simulink model "RL_sus_quarter_sim"  (R2025a)
settings: Solver=FixedStepAuto  StartTime=0.0  StopTime=20  FixedStep=0.001  RelTol=1e-3
model workspace (MAT data in the model file):
  G0 : Simulink.Parameter (value not decoded)
  Q_F : Simulink.Parameter (value not decoded)
  Q_dot_s : Simulink.Parameter (value not decoded)
  Q_dot_s_h : Simulink.Parameter (value not decoded)
  Q_dot_u : Simulink.Parameter (value not decoded)
  Q_flec : Simulink.Parameter (value not decoded)
  Q_flec_t : Simulink.Parameter (value not decoded)
  b_deflec : Simulink.Parameter (value not decoded)
  bump_height : Simulink.Parameter (value not decoded)
  bump_lenth : Simulink.Parameter (value not decoded)
  bump_start : Simulink.Parameter (value not decoded)
  f0 : Simulink.Parameter (value not decoded)
  kt : Simulink.Parameter (value not decoded)
  ms : Simulink.Parameter (value not decoded)
  n0 : Simulink.Parameter (value not decoded)
  n1 : Simulink.Parameter (value not decoded)
  omega_1 : Simulink.Parameter (value not decoded)
  omega_2 : Simulink.Parameter (value not decoded)
  omega_3 : Simulink.Parameter (value not decoded)
  omega_4 : Simulink.Parameter (value not decoded)
  ramp_height : Simulink.Parameter (value not decoded)
  ramp_lenth : Simulink.Parameter (value not decoded)
  ramp_start : Simulink.Parameter (value not decoded)
  sine_amp : Simulink.Parameter (value not decoded)
  sine_freq : Simulink.Parameter (value not decoded)
  u : Simulink.Parameter (value not decoded)
symbols that are objects in the model workspace (value not decoded): b_deflec, bump_height, bump_lenth, bump_start, f0, G0, kt, ms, n0, n1, omega_1, omega_2, omega_3, omega_4, Q_dot_s, Q_dot_s_h, Q_F, Q_flec, Q_flec_t, ramp_height, ramp_lenth, ramp_start, sine_amp, sine_freq
undefined symbols (not defined in the file): Ground, Hook, SH_ADD_new_as_as_xdef
libraries: fl_lib x250, nesl_utility x48, sharedTrackingLibrary x34, dspstat3 x18, simulink x3, deeplib x2, slpidlib x1
(part 12 of 12)

== system RL_sus_quarter_sim/Quarter_sys/Control/Y_1/IFEKF freq c/Subsystem/MATLAB Function2/IFEKF simple ==
  y : Inport
  Constant : Constant  Value=diag([0,0,0,0,1])
  Constant7 : Constant  Value=10  SampleTime=0.001
  Extended Kalman Filter1 : sharedTrackingLibrary/Extended Kalman Filter  StateTransitionFcn=IFEKF_tfcn_simp  HasStateTransitionJacobianFcn=on  StateTransitionJacobianFcn=IFEKF_jcob_fcn_simp  HasAdditiveProcessNoise=Additive  ProcessNoise=[0,0,1e-7,1e-10,0]  HasTimeVaryingProcessNoise=on  HasStateTransitionFcnExtraArgument=0  InitialState=[0;-1;0;-1;0.1*pi;]  InitialStateCovariance=[1e-1,1e-1,1e-1,1e-1,1e-5]  MeasurementFcn1=IFEKF_measure_fcn_simp  HasMeasurementJacobianFcn1=on  MeasurementJacobianFcn1=IFEKF_mea_jcob_fcn_simp  HasMeasurementEnablePort1=off  HasAdditiveMeasurementNoise1=Additive  MeasurementNoise1=0.0001  HasTimeVaryingMeasurementNoise1=on  HasMeasurementFcnExtraArgument1=0  HasMeasurementWrapping1=off  MeasurementFcn2=myMeasurementFcn  HasMeasurementJacobianFcn2=off  HasMeasurementEnablePort2=off  HasAdditiveMeasurementNoise2=Additive  MeasurementNoise2=1  HasTimeVaryingMeasurementNoise2=off  HasMeasurementFcnExtraArgument2=0  HasMeasurementWrapping2=off  MeasurementFcn3=myMeasurementFcn  HasMeasurementJacobianFcn3=off  HasMeasurementEnablePort3=off  HasAdditiveMeasurementNoise3=Additive  MeasurementNoise3=1  HasTimeVaryingMeasurementNoise3=off  HasMeasurementFcnExtraArgument3=0  HasMeasurementWrapping3=off  MeasurementFcn4=myMeasurementFcn  HasMeasurementJacobianFcn4=off  HasMeasurementEnablePort4=off  HasAdditiveMeasurementNoise4=Additive  MeasurementNoise4=1  HasTimeVaryingMeasurementNoise4=off  HasMeasurementFcnExtraArgument4=0  HasMeasurementWrapping4=off  MeasurementFcn5=myMeasurementFcn  HasMeasurementJacobianFcn5=off  HasMeasurementEnablePort5=off  HasAdditiveMeasurementNoise5=Additive  MeasurementNoise5=1  HasTimeVaryingMeasurementNoise5=off  HasMeasurementFcnExtraArgument5=0  HasMeasurementWrapping5=off  EnableMultirate=off  StateTransitionFcnSampleTime=1  MeasurementFcn1SampleTime=1  MeasurementFcn2SampleTime=1  MeasurementFcn3SampleTime=1  MeasurementFcn4SampleTime=1  MeasurementFcn5SampleTime=1  UseCurrentEstimator=off  OutputStateCovariance=on  DataType=double  SampleTime=0.001  NumberOfMeasurements=1
  Gain6 : Gain  Gain=1/2/pi
  Scope1 : Scope
      settings: ActiveDisplayYMinimum=-108223.31295  ActiveDisplayYMaximum=120159.3313  DataLoggingVariableName=ScopeData2
  Scope6 : Scope
      settings: ActiveDisplayYMinimum=-5.04517  ActiveDisplayYMaximum=3.95687  DataLoggingVariableName=ScopeData3
  Selector1 : Selector  InputPortWidth=5  IndexOptions=Index vector (dialog)  Indices=[1]  OutputSizes=1
  Selector8 : Selector  InputPortWidth=5  IndexOptions=Index vector (dialog)  Indices=[5]  OutputSizes=1
  x1hat : Outport
  P : Outport  Port=2
  debug : Outport  Port=3
  xhat_pred : Outport  Port=4
  y_residual : Outport  Port=5
  omega : Outport  Port=6
  wires:
  y/1 -> Extended Kalman Filter1/2
  Extended Kalman Filter1/2 -> P/1
  Constant7/1 -> Extended Kalman Filter1/3
  Constant/1 -> Extended Kalman Filter1/1
  Gain6/1 -> omega/1, Scope6/1
  Selector8/1 -> Gain6/1
  Selector1/1 -> x1hat/1
  Extended Kalman Filter1/1 -> Selector1/1, Selector8/1, Scope1/1

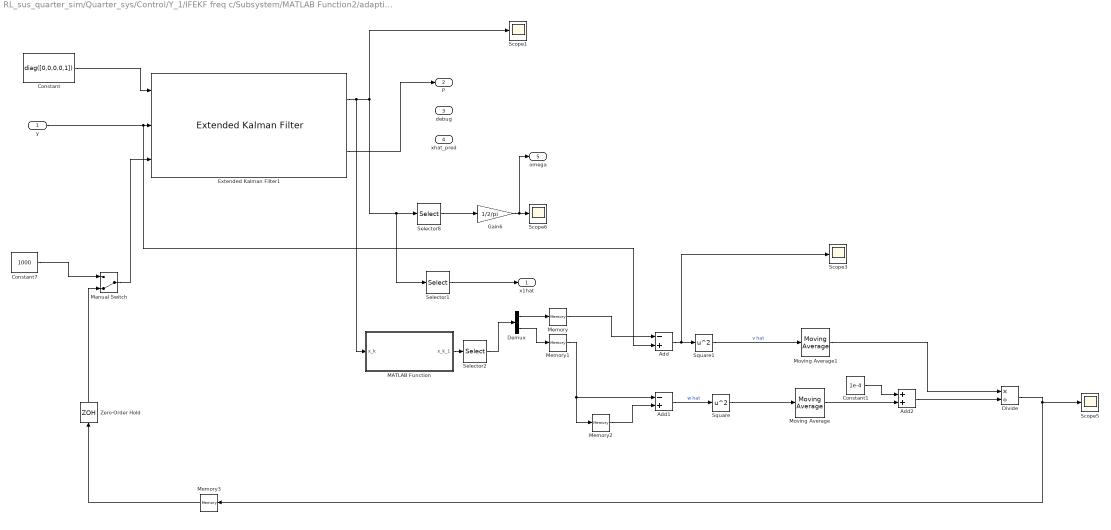
== system RL_sus_quarter_sim/Quarter_sys/Control/Y_1/IFEKF freq c/Subsystem/MATLAB Function2/adaptive IFEKF simple ==
  y : Inport
  Add : Sum  Inputs=-+
  Add1 : Sum  Inputs=-+
  Add2 : Sum
  Constant : Constant  Value=diag([0,0,0,0,1])
  Constant1 : Constant  Value=1e-4
  Constant7 : Constant  Value=1000  SampleTime=0.001
  Demux : Demux  Outputs=2
  Divide : Product  Inputs=*/
  Extended Kalman Filter1 : sharedTrackingLibrary/Extended Kalman Filter  StateTransitionFcn=IFEKF_tfcn_simp  HasStateTransitionJacobianFcn=on  StateTransitionJacobianFcn=IFEKF_jcob_fcn_simp  HasAdditiveProcessNoise=Additive  ProcessNoise=[0,0,1e-7,1e-10,0]  HasTimeVaryingProcessNoise=on  HasStateTransitionFcnExtraArgument=0  InitialState=[0;-1;0;-1;0.1*pi;]  InitialStateCovariance=[1e-1,1e-1,1e-1,1e-1,1e-5]  MeasurementFcn1=IFEKF_measure_fcn_simp  HasMeasurementJacobianFcn1=on  MeasurementJacobianFcn1=IFEKF_mea_jcob_fcn_simp  HasMeasurementEnablePort1=off  HasAdditiveMeasurementNoise1=Additive  MeasurementNoise1=0.0001  HasTimeVaryingMeasurementNoise1=on  HasMeasurementFcnExtraArgument1=0  HasMeasurementWrapping1=off  MeasurementFcn2=myMeasurementFcn  HasMeasurementJacobianFcn2=off  HasMeasurementEnablePort2=off  HasAdditiveMeasurementNoise2=Additive  MeasurementNoise2=1  HasTimeVaryingMeasurementNoise2=off  HasMeasurementFcnExtraArgument2=0  HasMeasurementWrapping2=off  MeasurementFcn3=myMeasurementFcn  HasMeasurementJacobianFcn3=off  HasMeasurementEnablePort3=off  HasAdditiveMeasurementNoise3=Additive  MeasurementNoise3=1  HasTimeVaryingMeasurementNoise3=off  HasMeasurementFcnExtraArgument3=0  HasMeasurementWrapping3=off  MeasurementFcn4=myMeasurementFcn  HasMeasurementJacobianFcn4=off  HasMeasurementEnablePort4=off  HasAdditiveMeasurementNoise4=Additive  MeasurementNoise4=1  HasTimeVaryingMeasurementNoise4=off  HasMeasurementFcnExtraArgument4=0  HasMeasurementWrapping4=off  MeasurementFcn5=myMeasurementFcn  HasMeasurementJacobianFcn5=off  HasMeasurementEnablePort5=off  HasAdditiveMeasurementNoise5=Additive  MeasurementNoise5=1  HasTimeVaryingMeasurementNoise5=off  HasMeasurementFcnExtraArgument5=0  HasMeasurementWrapping5=off  EnableMultirate=off  StateTransitionFcnSampleTime=1  MeasurementFcn1SampleTime=1  MeasurementFcn2SampleTime=1  MeasurementFcn3SampleTime=1  MeasurementFcn4SampleTime=1  MeasurementFcn5SampleTime=1  UseCurrentEstimator=off  OutputStateCovariance=on  DataType=double  SampleTime=0.001  NumberOfMeasurements=1
  Gain6 : Gain  Gain=1/2/pi
  MATLAB Function : MATLAB Function  TreatAsAtomicUnit=on
  Manual Switch : ManualSwitch  CurrentSetting=0
  Memory : Memory  InitialCondition=5
  Memory1 : Memory
  Memory2 : Memory  InitialCondition=1
  Memory3 : Memory  InitialCondition=10
  Moving Average : dspstat3/Moving Average  Method=Exponential weighting  ForgettingFactorPort=off  SpecifyWindowLength=off  WindowLength=100  OverlapLength=50  AllowArbitraryInputLength=on  ForgettingFactor=0.999  SimulateUsing=Interpreted execution
  Moving Average1 : dspstat3/Moving Average  Method=Exponential weighting  ForgettingFactorPort=off  SpecifyWindowLength=off  WindowLength=100  OverlapLength=50  AllowArbitraryInputLength=on  ForgettingFactor=0.999  SimulateUsing=Interpreted execution
  Scope{1,3,5..6} (4 alike) : Scope
      Scope1 settings: ActiveDisplayYMinimum=-108223.31295  ActiveDisplayYMaximum=120159.3313  DataLoggingVariableName=ScopeData3
      Scope3 settings: ActiveDisplayYMinimum=-5.93217  ActiveDisplayYMaximum=3.44712  DataLoggingVariableName=ScopeData4
      Scope5 settings: ActiveDisplayYMinimum=-180.87615  ActiveDisplayYMaximum=1627.8871  DataLoggingVariableName=ScopeData6
      Scope6 settings: ActiveDisplayYMinimum=-2.71822  ActiveDisplayYMaximum=5.24485  DataLoggingVariableName=ScopeData8
  Selector1 : Selector  InputPortWidth=5  IndexOptions=Index vector (dialog)  Indices=[1]  OutputSizes=1
  Selector2 : Selector  InputPortWidth=5  IndexOptions=Index vector (dialog)  Indices=[1 5]  OutputSizes=1
  Selector8 : Selector  InputPortWidth=5  IndexOptions=Index vector (dialog)  Indices=[5]  OutputSizes=1
  Square : Math  Operator=square
  Square1 : Math  Operator=square
  Zero-Order Hold : ZeroOrderHold  SampleTime=0.001
  x1hat : Outport
  P : Outport  Port=2
  debug : Outport  Port=3
  xhat_pred : Outport  Port=4
  omega : Outport  Port=5
  wires:
  Add1/1 -> Square/1  "w hat"
  Demux/2 -> Memory1/1
  Constant1/1 -> Add2/1
  Zero-Order Hold/1 -> Manual Switch/2
  Memory2/1 -> Add1/2
  Manual Switch/1 -> Extended Kalman Filter1/3
  MATLAB Function/1(x_k_1) -> Selector2/1
  Moving Average1/1 -> Divide/1
  Selector2/1 -> Demux/1
  Add2/1 -> Divide/2
  Constant/1 -> Extended Kalman Filter1/1
  Selector1/1 -> x1hat/1
  Moving Average/1 -> Add2/2
  Memory/1 -> Add/1
  Extended Kalman Filter1/1 -> MATLAB Function/1(x_k), Scope1/1, Selector8/1, Selector1/1
  y/1 -> Add/2, Extended Kalman Filter1/2
  Memory1/1 -> Add1/1, Memory2/1
  Square/1 -> Moving Average/1
  Square1/1 -> Moving Average1/1  "v hat"
  Extended Kalman Filter1/2 -> P/1
  Divide/1 -> Memory3/1, Scope5/1
  Selector8/1 -> Gain6/1
  Demux/1 -> Memory/1
  Add/1 -> Scope3/1, Square1/1
  Memory3/1 -> Zero-Order Hold/1
  Gain6/1 -> Scope6/1, omega/1
  Constant7/1 -> Manual Switch/1

== system RL_sus_quarter_sim/Quarter_sys/Control/Y_1/imp_force_RL_model/Subsystem/MATLAB Function2/EKF epsilon ==
  y : Inport
  epsilon : Inport  Port=2
  Constant : Constant  Value=diag([0,0,1,0])
  Constant7 : Constant  Value=500  SampleTime=0.001
  Extended Kalman Filter1 : sharedTrackingLibrary/Extended Kalman Filter  StateTransitionFcn=IFEKF_tfcn_ep  HasStateTransitionJacobianFcn=on  StateTransitionJacobianFcn=IFEKF_jcob_fcn_ep  HasAdditiveProcessNoise=Additive  ProcessNoise=[0,0,1e-7,1e-10]  HasTimeVaryingProcessNoise=on  HasStateTransitionFcnExtraArgument=1  InitialState=[0;-0.2;1*2*pi;0.2;]  InitialStateCovariance=[1e-1,1e-1,1e-1,1e-5]  MeasurementFcn1=IFEKF_measure_fcn_mod  HasMeasurementJacobianFcn1=on  MeasurementJacobianFcn1=IFEKF_mea_jcob_fcn_mod  HasMeasurementEnablePort1=off  HasAdditiveMeasurementNoise1=Additive  MeasurementNoise1=0.0001  HasTimeVaryingMeasurementNoise1=on  HasMeasurementFcnExtraArgument1=0  HasMeasurementWrapping1=off  MeasurementFcn2=myMeasurementFcn  HasMeasurementJacobianFcn2=off  HasMeasurementEnablePort2=off  HasAdditiveMeasurementNoise2=Additive  MeasurementNoise2=1  HasTimeVaryingMeasurementNoise2=off  HasMeasurementFcnExtraArgument2=0  HasMeasurementWrapping2=off  MeasurementFcn3=myMeasurementFcn  HasMeasurementJacobianFcn3=off  HasMeasurementEnablePort3=off  HasAdditiveMeasurementNoise3=Additive  MeasurementNoise3=1  HasTimeVaryingMeasurementNoise3=off  HasMeasurementFcnExtraArgument3=0  HasMeasurementWrapping3=off  MeasurementFcn4=myMeasurementFcn  HasMeasurementJacobianFcn4=off  HasMeasurementEnablePort4=off  HasAdditiveMeasurementNoise4=Additive  MeasurementNoise4=1  HasTimeVaryingMeasurementNoise4=off  HasMeasurementFcnExtraArgument4=0  HasMeasurementWrapping4=off  MeasurementFcn5=myMeasurementFcn  HasMeasurementJacobianFcn5=off  HasMeasurementEnablePort5=off  HasAdditiveMeasurementNoise5=Additive  MeasurementNoise5=1  HasTimeVaryingMeasurementNoise5=off  HasMeasurementFcnExtraArgument5=0  HasMeasurementWrapping5=off  EnableMultirate=off  StateTransitionFcnSampleTime=1  MeasurementFcn1SampleTime=1  MeasurementFcn2SampleTime=1  MeasurementFcn3SampleTime=1  MeasurementFcn4SampleTime=1  MeasurementFcn5SampleTime=1  UseCurrentEstimator=off  OutputStateCovariance=on  DataType=double  SampleTime=0.001  NumberOfMeasurements=1
  Gain6 : Gain  Gain=1/2/pi
  Scope6 : Scope
      settings: ActiveDisplayYMinimum=-0.3996  ActiveDisplayYMaximum=6.53697  DataLoggingVariableName=ScopeData2
  Selector1 : Selector  InputPortWidth=4  IndexOptions=Index vector (dialog)  Indices=[1]  OutputSizes=1
  Selector8 : Selector  InputPortWidth=4  IndexOptions=Index vector (dialog)  Indices=[3]  OutputSizes=1
  x1hat : Outport
  P : Outport  Port=2
  debug : Outport  Port=3
  xhat_pred : Outport  Port=4
  y_residual : Outport  Port=5
  omega : Outport  Port=6
  wires:
  y/1 -> Extended Kalman Filter1/3
  Extended Kalman Filter1/2 -> P/1
  Constant7/1 -> Extended Kalman Filter1/4
  epsilon/1 -> Extended Kalman Filter1/2
  Constant/1 -> Extended Kalman Filter1/1
  Gain6/1 -> omega/1, Scope6/1
  Selector8/1 -> Gain6/1
  Extended Kalman Filter1/1 -> Selector1/1, Selector8/1
  Selector1/1 -> x1hat/1

== system RL_sus_quarter_sim/Quarter_sys/Control/Y_1/imp_force_RL_model/Subsystem/MATLAB Function2/EKF simple Amp ==
  y : Inport
  epsilon : Inport  Port=2
  Constant5 : Constant  Value=0.1e-5
  Constant7 : Constant  Value=0.11  SampleTime=0.001
  Extended Kalman Filter1 : sharedTrackingLibrary/Extended Kalman Filter  StateTransitionFcn=IFEKF_tfcn_amp  HasStateTransitionJacobianFcn=on  StateTransitionJacobianFcn=IFEKF_jcob_fcn_amp  HasAdditiveProcessNoise=Additive  ProcessNoise=[0,0,1e-7,1e-10]  HasTimeVaryingProcessNoise=on  HasStateTransitionFcnExtraArgument=1  InitialState=[0;-0.5;2*pi;0.5;]  InitialStateCovariance=[1e-1,1e-1,1e-1,1e-5]  MeasurementFcn1=IFEKF_measure_fcn_amp  HasMeasurementJacobianFcn1=on  MeasurementJacobianFcn1=IFEKF_mea_jcob_fcn_amp  HasMeasurementEnablePort1=off  HasAdditiveMeasurementNoise1=Additive  MeasurementNoise1=0.0001  HasTimeVaryingMeasurementNoise1=on  HasMeasurementFcnExtraArgument1=0  HasMeasurementWrapping1=off  MeasurementFcn2=myMeasurementFcn  HasMeasurementJacobianFcn2=off  HasMeasurementEnablePort2=off  HasAdditiveMeasurementNoise2=Additive  MeasurementNoise2=1  HasTimeVaryingMeasurementNoise2=off  HasMeasurementFcnExtraArgument2=0  HasMeasurementWrapping2=off  MeasurementFcn3=myMeasurementFcn  HasMeasurementJacobianFcn3=off  HasMeasurementEnablePort3=off  HasAdditiveMeasurementNoise3=Additive  MeasurementNoise3=1  HasTimeVaryingMeasurementNoise3=off  HasMeasurementFcnExtraArgument3=0  HasMeasurementWrapping3=off  MeasurementFcn4=myMeasurementFcn  HasMeasurementJacobianFcn4=off  HasMeasurementEnablePort4=off  HasAdditiveMeasurementNoise4=Additive  MeasurementNoise4=1  HasTimeVaryingMeasurementNoise4=off  HasMeasurementFcnExtraArgument4=0  HasMeasurementWrapping4=off  MeasurementFcn5=myMeasurementFcn  HasMeasurementJacobianFcn5=off  HasMeasurementEnablePort5=off  HasAdditiveMeasurementNoise5=Additive  MeasurementNoise5=1  HasTimeVaryingMeasurementNoise5=off  HasMeasurementFcnExtraArgument5=0  HasMeasurementWrapping5=off  EnableMultirate=off  StateTransitionFcnSampleTime=1  MeasurementFcn1SampleTime=1  MeasurementFcn2SampleTime=1  MeasurementFcn3SampleTime=1  MeasurementFcn4SampleTime=1  MeasurementFcn5SampleTime=1  UseCurrentEstimator=off  OutputStateCovariance=on  DataType=double  SampleTime=0.001  NumberOfMeasurements=1
  Gain6 : Gain  Gain=1/2/pi
  MATLAB Function : MATLAB Function
  Scope1 : Scope
      settings: ActiveDisplayYMinimum=-1.3479  ActiveDisplayYMaximum=7.13108  DataLoggingVariableName=ScopeData7
  Scope6 : Scope
      settings: ActiveDisplayYMinimum=0.9999988  ActiveDisplayYMaximum=1.0000001
  Selector1 : Selector  InputPortWidth=4  IndexOptions=Index vector (dialog)  Indices=[1]  OutputSizes=1
  Selector8 : Selector  InputPortWidth=4  IndexOptions=Index vector (dialog)  Indices=[3]  OutputSizes=1
  x1hat : Outport
  P : Outport  Port=2
  debug : Outport  Port=3
  xhat_pred : Outport  Port=4
  y_residual : Outport  Port=5
  omega : Outport  Port=6
  wires:
  epsilon/1 -> Extended Kalman Filter1/2
  Constant7/1 -> Extended Kalman Filter1/4
  Constant5/1 -> MATLAB Function/1(gamma)
  Extended Kalman Filter1/2 -> P/1
  y/1 -> Extended Kalman Filter1/3
  MATLAB Function/1(y) -> Extended Kalman Filter1/1
  Extended Kalman Filter1/1 -> Selector1/1, Selector8/1, Scope1/1
  Selector8/1 -> Gain6/1
  Gain6/1 -> omega/1, Scope6/1
  Selector1/1 -> x1hat/1

== system RL_sus_quarter_sim/Quarter_sys/Control/Y_1/imp_force_RL_model/Subsystem/MATLAB Function2/IFEKF simple ==
  y : Inport
  Constant : Constant  Value=diag([0,0,0,0,1])
  Constant7 : Constant  Value=10  SampleTime=0.001
  Extended Kalman Filter1 : sharedTrackingLibrary/Extended Kalman Filter  StateTransitionFcn=IFEKF_tfcn_simp  HasStateTransitionJacobianFcn=on  StateTransitionJacobianFcn=IFEKF_jcob_fcn_simp  HasAdditiveProcessNoise=Additive  ProcessNoise=[0,0,1e-7,1e-10,0]  HasTimeVaryingProcessNoise=on  HasStateTransitionFcnExtraArgument=0  InitialState=[0;-1;0;-1;0.1*pi;]  InitialStateCovariance=[1e-1,1e-1,1e-1,1e-1,1e-5]  MeasurementFcn1=IFEKF_measure_fcn_simp  HasMeasurementJacobianFcn1=on  MeasurementJacobianFcn1=IFEKF_mea_jcob_fcn_simp  HasMeasurementEnablePort1=off  HasAdditiveMeasurementNoise1=Additive  MeasurementNoise1=0.0001  HasTimeVaryingMeasurementNoise1=on  HasMeasurementFcnExtraArgument1=0  HasMeasurementWrapping1=off  MeasurementFcn2=myMeasurementFcn  HasMeasurementJacobianFcn2=off  HasMeasurementEnablePort2=off  HasAdditiveMeasurementNoise2=Additive  MeasurementNoise2=1  HasTimeVaryingMeasurementNoise2=off  HasMeasurementFcnExtraArgument2=0  HasMeasurementWrapping2=off  MeasurementFcn3=myMeasurementFcn  HasMeasurementJacobianFcn3=off  HasMeasurementEnablePort3=off  HasAdditiveMeasurementNoise3=Additive  MeasurementNoise3=1  HasTimeVaryingMeasurementNoise3=off  HasMeasurementFcnExtraArgument3=0  HasMeasurementWrapping3=off  MeasurementFcn4=myMeasurementFcn  HasMeasurementJacobianFcn4=off  HasMeasurementEnablePort4=off  HasAdditiveMeasurementNoise4=Additive  MeasurementNoise4=1  HasTimeVaryingMeasurementNoise4=off  HasMeasurementFcnExtraArgument4=0  HasMeasurementWrapping4=off  MeasurementFcn5=myMeasurementFcn  HasMeasurementJacobianFcn5=off  HasMeasurementEnablePort5=off  HasAdditiveMeasurementNoise5=Additive  MeasurementNoise5=1  HasTimeVaryingMeasurementNoise5=off  HasMeasurementFcnExtraArgument5=0  HasMeasurementWrapping5=off  EnableMultirate=off  StateTransitionFcnSampleTime=1  MeasurementFcn1SampleTime=1  MeasurementFcn2SampleTime=1  MeasurementFcn3SampleTime=1  MeasurementFcn4SampleTime=1  MeasurementFcn5SampleTime=1  UseCurrentEstimator=off  OutputStateCovariance=on  DataType=double  SampleTime=0.001  NumberOfMeasurements=1
  Gain6 : Gain  Gain=1/2/pi
  Scope1 : Scope
      settings: ActiveDisplayYMinimum=-108223.31295  ActiveDisplayYMaximum=120159.3313  DataLoggingVariableName=ScopeData2
  Scope6 : Scope
      settings: ActiveDisplayYMinimum=-5.04517  ActiveDisplayYMaximum=3.95687  DataLoggingVariableName=ScopeData3
  Selector1 : Selector  InputPortWidth=5  IndexOptions=Index vector (dialog)  Indices=[1]  OutputSizes=1
  Selector8 : Selector  InputPortWidth=5  IndexOptions=Index vector (dialog)  Indices=[5]  OutputSizes=1
  x1hat : Outport
  P : Outport  Port=2
  debug : Outport  Port=3
  xhat_pred : Outport  Port=4
  y_residual : Outport  Port=5
  omega : Outport  Port=6
  wires:
  y/1 -> Extended Kalman Filter1/2
  Extended Kalman Filter1/2 -> P/1
  Constant7/1 -> Extended Kalman Filter1/3
  Constant/1 -> Extended Kalman Filter1/1
  Gain6/1 -> omega/1, Scope6/1
  Selector8/1 -> Gain6/1
  Selector1/1 -> x1hat/1
  Extended Kalman Filter1/1 -> Selector1/1, Selector8/1, Scope1/1

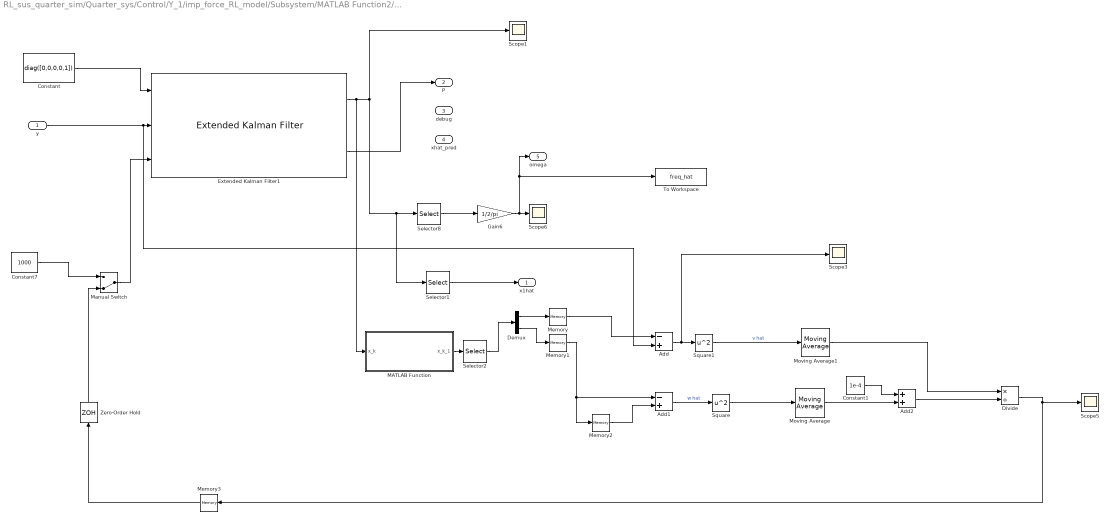
== system RL_sus_quarter_sim/Quarter_sys/Control/Y_1/imp_force_RL_model/Subsystem/MATLAB Function2/adaptive IFEKF simple ==
  y : Inport
  Add : Sum  Inputs=-+
  Add1 : Sum  Inputs=-+
  Add2 : Sum
  Constant : Constant  Value=diag([0,0,0,0,1])
  Constant1 : Constant  Value=1e-4
  Constant7 : Constant  Value=1000  SampleTime=0.001
  Demux : Demux  Outputs=2
  Divide : Product  Inputs=*/
  Extended Kalman Filter1 : sharedTrackingLibrary/Extended Kalman Filter  StateTransitionFcn=IFEKF_tfcn_simp  HasStateTransitionJacobianFcn=on  StateTransitionJacobianFcn=IFEKF_jcob_fcn_simp  HasAdditiveProcessNoise=Additive  ProcessNoise=[0,0,1e-7,1e-10,0]  HasTimeVaryingProcessNoise=on  HasStateTransitionFcnExtraArgument=0  InitialState=[0;-1;0;-1;0.1*pi;]  InitialStateCovariance=[1e-1,1e-1,1e-1,1e-1,1e-5]  MeasurementFcn1=IFEKF_measure_fcn_simp  HasMeasurementJacobianFcn1=on  MeasurementJacobianFcn1=IFEKF_mea_jcob_fcn_simp  HasMeasurementEnablePort1=off  HasAdditiveMeasurementNoise1=Additive  MeasurementNoise1=0.0001  HasTimeVaryingMeasurementNoise1=on  HasMeasurementFcnExtraArgument1=0  HasMeasurementWrapping1=off  MeasurementFcn2=myMeasurementFcn  HasMeasurementJacobianFcn2=off  HasMeasurementEnablePort2=off  HasAdditiveMeasurementNoise2=Additive  MeasurementNoise2=1  HasTimeVaryingMeasurementNoise2=off  HasMeasurementFcnExtraArgument2=0  HasMeasurementWrapping2=off  MeasurementFcn3=myMeasurementFcn  HasMeasurementJacobianFcn3=off  HasMeasurementEnablePort3=off  HasAdditiveMeasurementNoise3=Additive  MeasurementNoise3=1  HasTimeVaryingMeasurementNoise3=off  HasMeasurementFcnExtraArgument3=0  HasMeasurementWrapping3=off  MeasurementFcn4=myMeasurementFcn  HasMeasurementJacobianFcn4=off  HasMeasurementEnablePort4=off  HasAdditiveMeasurementNoise4=Additive  MeasurementNoise4=1  HasTimeVaryingMeasurementNoise4=off  HasMeasurementFcnExtraArgument4=0  HasMeasurementWrapping4=off  MeasurementFcn5=myMeasurementFcn  HasMeasurementJacobianFcn5=off  HasMeasurementEnablePort5=off  HasAdditiveMeasurementNoise5=Additive  MeasurementNoise5=1  HasTimeVaryingMeasurementNoise5=off  HasMeasurementFcnExtraArgument5=0  HasMeasurementWrapping5=off  EnableMultirate=off  StateTransitionFcnSampleTime=1  MeasurementFcn1SampleTime=1  MeasurementFcn2SampleTime=1  MeasurementFcn3SampleTime=1  MeasurementFcn4SampleTime=1  MeasurementFcn5SampleTime=1  UseCurrentEstimator=off  OutputStateCovariance=on  DataType=double  SampleTime=0.001  NumberOfMeasurements=1
  Gain6 : Gain  Gain=1/2/pi
  MATLAB Function : MATLAB Function  TreatAsAtomicUnit=on
  Manual Switch : ManualSwitch  CurrentSetting=0
  Memory : Memory  InitialCondition=5
  Memory1 : Memory
  Memory2 : Memory  InitialCondition=1
  Memory3 : Memory  InitialCondition=10
  Moving Average : dspstat3/Moving Average  Method=Exponential weighting  ForgettingFactorPort=off  SpecifyWindowLength=off  WindowLength=100  OverlapLength=50  AllowArbitraryInputLength=on  ForgettingFactor=0.999  SimulateUsing=Interpreted execution
  Moving Average1 : dspstat3/Moving Average  Method=Exponential weighting  ForgettingFactorPort=off  SpecifyWindowLength=off  WindowLength=100  OverlapLength=50  AllowArbitraryInputLength=on  ForgettingFactor=0.999  SimulateUsing=Interpreted execution
  Scope{1,3,5..6} (4 alike) : Scope
      Scope1 settings: ActiveDisplayYMinimum=-5.9836760801118811E+37  ActiveDisplayYMaximum=5.3206752918754988E+37  DataLoggingVariableName=ScopeData3
      Scope3 settings: ActiveDisplayYMinimum=-5.93217  ActiveDisplayYMaximum=3.44712  DataLoggingVariableName=ScopeData4
      Scope5 settings: ActiveDisplayYMinimum=-182.59879  ActiveDisplayYMaximum=1643.39044  DataLoggingVariableName=ScopeData6
      Scope6 settings: ActiveDisplayYMinimum=-3.1891  ActiveDisplayYMaximum=3.16461  DataLoggingVariableName=ScopeData8
  Selector1 : Selector  InputPortWidth=5  IndexOptions=Index vector (dialog)  Indices=[1]  OutputSizes=1
  Selector2 : Selector  InputPortWidth=5  IndexOptions=Index vector (dialog)  Indices=[1 5]  OutputSizes=1
  Selector8 : Selector  InputPortWidth=5  IndexOptions=Index vector (dialog)  Indices=[5]  OutputSizes=1
  Square : Math  Operator=square
  Square1 : Math  Operator=square
  To Workspace : ToWorkspace  VariableName=freq_hat  SampleTime=-1
  Zero-Order Hold : ZeroOrderHold  SampleTime=0.001
  x1hat : Outport
  P : Outport  Port=2
  debug : Outport  Port=3
  xhat_pred : Outport  Port=4
  omega : Outport  Port=5
  wires:
  Add1/1 -> Square/1  "w hat"
  Demux/2 -> Memory1/1
  Constant1/1 -> Add2/1
  Zero-Order Hold/1 -> Manual Switch/2
  Memory2/1 -> Add1/2
  Manual Switch/1 -> Extended Kalman Filter1/3
  MATLAB Function/1(x_k_1) -> Selector2/1
  Moving Average1/1 -> Divide/1
  Selector2/1 -> Demux/1
  Add2/1 -> Divide/2
  Constant/1 -> Extended Kalman Filter1/1
  Selector1/1 -> x1hat/1
  Moving Average/1 -> Add2/2
  Memory/1 -> Add/1
  Extended Kalman Filter1/1 -> MATLAB Function/1(x_k), Scope1/1, Selector8/1, Selector1/1
  y/1 -> Add/2, Extended Kalman Filter1/2
  Memory1/1 -> Add1/1, Memory2/1
  Square/1 -> Moving Average/1
  Square1/1 -> Moving Average1/1  "v hat"
  Extended Kalman Filter1/2 -> P/1
  Divide/1 -> Memory3/1, Scope5/1
  Selector8/1 -> Gain6/1
  Demux/1 -> Memory/1
  Add/1 -> Scope3/1, Square1/1
  Memory3/1 -> Zero-Order Hold/1
  Gain6/1 -> Scope6/1, To Workspace/1, omega/1
  Constant7/1 -> Manual Switch/1

== matlab function RL_sus_quarter_sim/road_profile/gp/MATLAB Function ==
  data: X input; u output; gp_sample input; x input
function u = u_fn(X, gp_sample, x)
    u = interp1(X, gp_sample, x, 'linear', 'extrap');
end

== matlab function RL_sus_quarter_sim/Quarter_sys/Control/Y_1/SH_ADD_new_as_as_xdef^2/2nd_FS_adef_vs/MATLAB Function1 ==
  data: as input; xdef input; y output; alpha input; ks input; ms input; cs input
function y = fcn(as,xdef,alpha,ks,ms,cs)

H2 = (cs^4*alpha^4 + (2*cs^2*ks^2)*alpha^2 + ks^4)/(ms^4*alpha^2);
y = xdef^4/as^2* alpha^2 * H2;

end

== matlab function RL_sus_quarter_sim/Quarter_sys/Control/Y_1/IFEKF freq bkkcc/Subsystem/MATLAB Function2/EKF simple Amp/MATLAB Function ==
  data: gamma input; y output size=[4,4]
function y = fcn(gamma)
% u = [0;0;gamma;1];
u = [0;0;1;gamma];
y = diag(u);
end

== matlab function RL_sus_quarter_sim/Quarter_sys/Control/Y_1/IFEKF freq bkkcc/Subsystem/MATLAB Function2/adaptive IFEKF simple/MATLAB Function ==
  data: x_k input; x_k_1 output
function x_k_1 = IFEKF_tfcn_simp(x_k)
x_k_1 = zeros(5,1);
dt = 0.001;
x_k_1(1) = 2*cos(x_k(5)*dt) * x_k(1) - x_k(2) ;
x_k_1(2) = x_k(1);
x_k_1(3) = 2*cos(x_k(5)*dt) * x_k(3) - x_k(4);
x_k_1(4) = x_k(3);
x_k_1(5) = x_k(5);
 
end

== stateflow chart RL_sus_quarter_sim/Quarter_sys/Control/Y_1/IFEKF freq bkkcc/Subsystem/Chart ==
  state L2
    entry:count = 0;
    level = 2;
    during:count = count+1;
    level = 2;
  state L1
    entry:count = 0;
    level = 1;
    during:count = count+1;
    level = 1;
  (default) -> L1
  L1 -> L2 : [freq > (FS1+0.1)&&freq<(FS2-0.1)&&count>=100]
  L2 -> L1 : [(freq<(FS1-0.1)&&count>=100)||(freq>(FS2+0.1)&&count>=100)]
  data: freq input; level output; FS1 input; FS2 input; data local; count local

== stateflow chart RL_sus_quarter_sim/Quarter_sys/Control/Y_1/imp_force_RL_model/Subsystem/Chart ==
  state L2
    entry:count = 0;
    level = 2;
    during:count = count+1;
    level = 2;
  state L1
    entry:count = 0;
    level = 1;
    during:count = count+1;
    level = 1;
  (default) -> L1
  L1 -> L2 : [freq > (FS1+0.1)&&freq<(FS2-0.1)&&count>=100]
  L2 -> L1 : [(freq<(FS1-0.1)&&count>=100)||(freq>(FS2+0.1)&&count>=100)]
  data: freq input; level output; FS1 input; FS2 input; data local; count local

== matlab function RL_sus_quarter_sim/Quarter_sys/Control/Y_1/IFEKF SHADD/Subsystem/MATLAB Function ==
  data: u input; FS_1 input; y output; FS_2 input; FS_3 input
function y = fcn(u,FS_1,FS_2,FS_3)

    % if u < FS_1
    %     y = 3;
    % elseif u >= FS_1 && u < FS_2
    %     y = 1;
    % elseif u >= FS_2 && u < FS_3
    %     y = 2;
    % else
    %     y = 1;
    % end


    if u < FS_1
        y = 1;
    else
        y = 2;
    end
end

== matlab function RL_sus_quarter_sim/Quarter_sys/Control/Y_1/freq semi/Subsystem/2nd_FS1/MATLAB Function1 ==
  data: au input; y output; alpha input; ks input; ms input; cs input
function y = fcn(au,alpha,ks,ms,cs)

y = au^2 * (ks^2 + alpha^2 * cs^2)/((ks-alpha^2*ms)^2 + alpha^2 * cs^2);
end

== stateflow chart RL_sus_quarter_sim/Quarter_sys/Control/Y_1/freq semi/Subsystem/Chart ==
  state Mid_freq
    entry:
    Select = 2;
    during:
    Select = 2;
  state High_freq
    entry:
    Select = 3;
    during:
    Select = 3;
  state Low_freq
    entry:
    Select = 1;
    during:
    Select = 1;
  (default) -> High_freq
  Mid_freq -> High_freq [order 1] : [FS_2>0]
  High_freq -> Mid_freq [order 1] : [(FS_2<0)&&(FS_1 >0)]
  High_freq -> Mid_freq [commented out] : [(FS_2<0)&&(FS_1 ==0)]
  Low_freq -> Mid_freq [order 1] : [(FS_2<0)&&FS_1 >0]
  Mid_freq -> Low_freq [order 2] : [FS_1<0]
  High_freq -> Low_freq [order 2] : [FS_1<0]
  Low_freq -> High_freq [order 2] : [FS_2>0]
  data: FS_1 input; FS_2 input; Select output

== matlab function RL_sus_quarter_sim/Quarter_sys/Control/Y_1/Freq_imp1/Subsystem/2nd_FS/MATLAB Function1 ==
  data: au input; y output; alpha input; ks input; ms input; cs input
function y = fcn(au,alpha,ks,ms,cs)

y = au^2 * (ks^2 + alpha^2 * cs^2)/((ks-alpha^2*ms)^2 + alpha^2 * cs^2);
end

== matlab function RL_sus_quarter_sim/Quarter_sys/Control/Y_1/Freq_imp1/Subsystem/FS1/MATLAB Function1 ==
  data: au input; y output; alpha input; ks input; ms input; cs input
function y = fcn(au,alpha,ks,ms,cs)

y = au^2 * (ks^2 + alpha^2 * cs^2)/((ks-alpha^2*ms)^2 + alpha^2 * cs^2);
end

== stateflow chart RL_sus_quarter_sim/Quarter_sys/Control/Y_1/Freq_imp1/Subsystem/Chart ==
  state Mid_freq
    entry:
    Select = 2;
    during:
    Select = 2;
  state High_freq
    entry:
    Select = 3;
    during:
    Select = 3;
  state Low_freq
    entry:
    Select = 1;
    during:
    Select = 1;
  (default) -> High_freq
  Mid_freq -> High_freq [order 1] : [FS_2>0]
  High_freq -> Mid_freq [order 1] : [(FS_2<0)&&(FS_1 >0)]
  High_freq -> Mid_freq [commented out] : [(FS_2<0)&&(FS_1 ==0)]
  Low_freq -> Mid_freq [order 1] : [(FS_2<0)&&FS_1 >0]
  Mid_freq -> Low_freq [order 2] : [FS_1<0]
  High_freq -> Low_freq [order 2] : [FS_1<0]
  Low_freq -> High_freq [order 2] : [FS_2>0]
  data: FS_1 input; FS_2 input; Select output

== matlab function RL_sus_quarter_sim/Quarter_sys/Control/Y_1/SH_ADD_new_FS/MATLAB Function ==
  data: as input; y output; vs input; vdef input; alpha input
function y = fcn(as,vs,vdef,alpha)
cs =1000;
ks = 20000;
ms = 400;

H_alpha = (cs^2*alpha^2+ks^2)/(ms^2*alpha^2);
    if (vdef^2*H_alpha - alpha^2 * vs^2)<=0
        if vs * vdef >0
            y = 1;
        else
            y = 0;
        end
    else
        if as * vdef >0
            y = 1;
        else
            y = 0;
        end
    end

end

== matlab function RL_sus_quarter_sim/Quarter_sys/Control/Y_1/IFEKF SHADD/Subsystem/MATLAB Function2/EKF simple Amp/MATLAB Function ==
  data: gamma input; y output size=[4,4]
function y = fcn(gamma)
% u = [0;0;gamma;1];
u = [0;0;1;gamma];
y = diag(u);
end

== matlab function RL_sus_quarter_sim/Quarter_sys/Control/Y_1/IFEKF SHADD/Subsystem/MATLAB Function2/adaptive IFEKF simple/MATLAB Function ==
  data: x_k input; x_k_1 output
function x_k_1 = IFEKF_tfcn_simp(x_k)
x_k_1 = zeros(5,1);
dt = 0.001;
x_k_1(1) = 2*cos(x_k(5)*dt) * x_k(1) - x_k(2) ;
x_k_1(2) = x_k(1);
x_k_1(3) = 2*cos(x_k(5)*dt) * x_k(3) - x_k(4);
x_k_1(4) = x_k(3);
x_k_1(5) = x_k(5);
 
end

== matlab function RL_sus_quarter_sim/Quarter_sys/Control/Y_1/IFEKF freq c/Subsystem/MATLAB Function ==
  data: u input; FS_1 input; y output; FS_2 input; FS_3 input
function y = fcn(u,FS_1,FS_2,FS_3)

    if u < FS_1
        y = 1;
    elseif u >= FS_1 && u < FS_2
        y = 2;
    elseif u >= FS_2 && u < FS_3
        y = 3;
    else
        y = 4;
    end


    % if u < FS_1
    %     y = 1;
    % else
    %     y = 2;
    % end
end

== matlab function RL_sus_quarter_sim/Quarter_sys/Control/Y_1/freq semi/Subsystem/1st_FS1 ==
  data: as input; y output; vs input; alpha1 input
function y = fcn(as,vs,alpha1)
    y = (as^2 - alpha1^2 * vs^2);
      
end

== matlab function RL_sus_quarter_sim/Quarter_sys/Control/Y_1/SH_ADD_new_as_au_xdef_vdef/2nd_FS_adef_vs/MATLAB Function1 ==
  data: xdef input; vdef input; y output; alpha input; ks input; ms input; cs input
function y = fcn(xdef,vdef,alpha,ks,ms,cs)

H2 = ((cs^2*ms^2)*alpha^6 + (cs^4 - 2*cs^2*ks*ms + ks^2*ms^2)*alpha^4 + (2*cs^2*ks^2 - 2*ks^3*ms)*alpha^2 + ks^4)/(ms^4*alpha^4);
y = xdef^2 * vdef^2 * alpha^2 * H2;

end

== matlab function RL_sus_quarter_sim/Quarter_sys/Control/Y_1/SH_ADD_new_au_vs/2nd_FS/MATLAB Function1 ==
  data: au input; y output; alpha input; ks input; ms input; cs input
function y = fcn(au,alpha,ks,ms,cs)

y = au^2 * (ks^2 + alpha^2 * cs^2)/((ks-alpha^2*ms)^2 + alpha^2 * cs^2);
end

== stateflow chart RL_sus_quarter_sim/Quarter_sys/Control/Y_1/imp_force_RL_model/Subsystem/Chart1 ==
  state L1
    entry:count = 0;
    level = 1;
    during:count = count+1;
    level = 1;
  state L2
    entry:count = 0;
    level = 2;
    during:count = count+1;
    level = 2;
  state L3
    entry:count = 0;
    level = 3;
    during:count = count+1;
    level = 3;
  state L4
    entry:count = 0;
    level = 4;
    during:count = count+1;
    level = 4;
  state L5
    entry:count = 0;
    level = 5;
    during:count = count+1;
    level = 5;
  state L6
    entry:count = 0;
    level = 6;
    during:count = count+1;
    level = 6;
  state L7
    entry:count = 0;
    level = 7;
    during:count = count+1;
    level = 7;
  (default) -> L1
  L1 -> L2 : [freq > (FS1+0.1)&&freq < (FS2-0.1)&&count>=200]
  L6 -> L7 [order 2] : [freq > (FS6+0.1)&&count>=100]
  L2 -> L1 [order 2] : [(freq<(FS1-0.1)&&count>=200)]
  L2 -> L3 [order 1] : [freq > (FS2+0.1)&&freq<(FS3-0.1)&&count>=100]
  L3 -> L4 [order 1] : [freq > (FS3+0.1)&&freq<(FS4-0.1)&&count>=100]
  L4 -> L5 [order 1] : [freq > (FS4+0.1)&&freq<(FS5-0.1)&&count>=100]
  L5 -> L6 [order 2] : [freq > (FS5+0.1)&&freq<(FS6-0.1)&&count>=100]
  L3 -> L2 [order 2] : [freq > (FS1+0.1)&&freq < (FS2-0.1)&&count>=100]
  L7 -> L6 : [freq > (FS5+0.1)&&freq<(FS6-0.1)&&count>=100]
  L5 -> L4 [order 1] : [freq > (FS3+0.1)&&freq<(FS4-0.1)&&count>=100]
  L6 -> L5 [order 1] : [freq > (FS4+0.1)&&freq<(FS5-0.1)&&count>=100]
  L4 -> L3 [order 2] : [freq > (FS2+0.1)&&freq<(FS3-0.1)&&count>=100]
  data: freq input; level output; FS3 constant double =7; count local; FS1 constant double =0.85; FS2 constant double =2.6; FS4 constant double =10; FS5 constant double =12.3; FS6 constant double =13.9

== matlab function RL_sus_quarter_sim/Quarter_sys/Control/Y_1/IFEKF Select c/Subsystem/MATLAB Function ==
  data: u input; FS_1 input; y output; FS_2 input
function y = fcn(u,FS_1,FS_2)

    if u < FS_1
        y = 1;
    elseif u >= FS_1 && u < FS_2
        y = 2;
    else
        y = 3;
    end
end

== matlab function RL_sus_quarter_sim/Quarter_sys/Control/Y_1/IFEKF Select c/Subsystem/MATLAB Function2/EKF simple Amp/MATLAB Function ==
  data: gamma input; y output size=[4,4]
function y = fcn(gamma)
% u = [0;0;gamma;1];
u = [0;0;1;gamma];
y = diag(u);
end

== matlab function RL_sus_quarter_sim/Subsystem1/Subsystem1/MATLAB Function4 ==
  data: t input; signal output
function signal = generate_chirp_signal(t)
    % 输入参数：
    % t: 单个时间点（标量）
    % 输出参数：
    % signal: 对应时间点的频率变化正弦信号值

    % 持久变量，用于存储上一次调用函数时的相位和时间
    persistent phase_prev t_prev;

    % 初始化持久变量
    if isempty(phase_prev)
        phase_prev = 0;
        t_prev = 0;
    end

    % 计算瞬时频率
    if t < 5
        % 0-5秒，频率从1Hz线性增加到3Hz
        freq = 1 + (3-1)*(t/5);
    elseif t < 10 && t >= 5
        % 5-10秒，频率保持3Hz
        freq = 3;
    elseif t < 15 && t >= 10
        % 10-15秒，频率从3Hz线性减小到1Hz
        freq = 3 - (3-1)*((t-10)/5);
    else
        freq = 1;
    end

    % 计算相位（频率的积分）
    % 使用梯形法近似积分
    delta_t = t - t_prev;
    phase = phase_prev + 2 * pi * freq * delta_t;

    % 更新持久变量
    phase_prev = phase;
    t_prev = t;

    % 生成正弦信号
    signal = sin(phase);
end

== matlab function RL_sus_quarter_sim/Subsystem1/Subsystem2/MATLAB Function3 ==
  data: t input; signal output
function signal = generate_chirp_signal(t)
    % 输入参数：
    % t: 单个时间点（标量）
    % 输出参数：
    % signal: 对应时间点的频率变化正弦信号值

    % 持久变量，用于存储上一次调用函数时的相位和时间
    persistent phase_prev t_prev;

    % 初始化持久变量
    if isempty(phase_prev)
        phase_prev = 0;
        t_prev = 0;
    end

    % 计算瞬时频率
    if t < 5
        % 0-5秒，频率从1Hz线性增加到3Hz
        freq = 1 + (3-1)*(t/5);
    elseif t < 10 && t >= 5
        % 5-10秒，频率保持3Hz
        freq = 3;
    elseif t < 15 && t >= 10
        % 10-15秒，频率从3Hz线性减小到1Hz
        freq = 3 - (3-1)*((t-10)/5);
    else
        freq = 1;
    end

    % 计算相位（频率的积分）
    % 使用梯形法近似积分
    delta_t = t - t_prev;
    phase = phase_prev + 2 * pi * freq * delta_t;

    % 更新持久变量
    phase_prev = phase;
    t_prev = t;

    % 计算时变幅值（示例：幅值从1线性增加到2，再减小到1）
    if t < 5
        amplitude = 1 + (5-1)*(t/5); % 0-5秒，幅值从1增加到2
    elseif t < 10 && t >= 5
        amplitude = 5; % 5-10秒，幅值保持2
    elseif t < 15 && t >= 10
        amplitude = 5 - (5-1)*((t-10)/5); % 10-15秒，幅值从2减小到1
    elseif t < 25 && t >= 15
        amplitude = 1;
    else
        amplitude = 1 - 0.05 * (t - 25);
    end

    % 生成正弦信号
    signal = amplitude * sin(phase);
end

== matlab function RL_sus_quarter_sim/Quarter_sys/Control/Y_1/IFEKF freq b/Subsystem/MATLAB Function ==
  data: u input; FS_1 input; y output; FS_2 input; FS_3 input
function y = fcn(u,FS_1,FS_2,FS_3)

    if u < FS_1
        y = 3;
    elseif u >= FS_1 && u < FS_2
        y = 1;
    elseif u >= FS_2 && u < FS_3
        y = 2;
    else
        y = 1;
    end
end

== matlab function RL_sus_quarter_sim/Quarter_sys/Control/Y_1/IFEKF freq b/Subsystem/MATLAB Function2/EKF simple Amp/MATLAB Function ==
  data: gamma input; y output size=[4,4]
function y = fcn(gamma)
% u = [0;0;gamma;1];
u = [0;0;1;gamma];
y = diag(u);
end

== matlab function RL_sus_quarter_sim/Quarter_sys/Control/Y_1/SH_ADD_new_xdef_vs/2nd_FS_adef_vs/MATLAB Function1 ==
  data: au input; y output; alpha input; ks input; ms input; cs input
function y = fcn(au,alpha,ks,ms,cs)

y = au^2 * (ks^2 + alpha^2 * cs^2)/((alpha^2*ms)^2);
end

== matlab function RL_sus_quarter_sim/Quarter_sys/Control/Y_1/IFEKF Select c/Subsystem/MATLAB Function2/adaptive IFEKF simple/MATLAB Function ==
  data: x_k input; x_k_1 output
function x_k_1 = IFEKF_tfcn_simp(x_k)
x_k_1 = zeros(5,1);
dt = 0.001;
x_k_1(1) = 2*cos(x_k(5)*dt) * x_k(1) - x_k(2) ;
x_k_1(2) = x_k(1);
x_k_1(3) = 2*cos(x_k(5)*dt) * x_k(3) - x_k(4);
x_k_1(4) = x_k(3);
x_k_1(5) = x_k(5);
 
end

== matlab function RL_sus_quarter_sim/Quarter_sys/Control/Y_1/imp_force_RL_model/Subsystem/MATLAB Function2/EKF simple Amp/MATLAB Function ==
  data: gamma input; y output size=[4,4]
function y = fcn(gamma)
% u = [0;0;gamma;1];
u = [0;0;1;gamma];
y = diag(u);
end

== matlab function RL_sus_quarter_sim/Quarter_sys/Control/Y_1/IFEKF freq b/Subsystem/MATLAB Function2/adaptive IFEKF simple/MATLAB Function ==
  data: x_k input; x_k_1 output
function x_k_1 = IFEKF_tfcn_simp(x_k)
x_k_1 = zeros(5,1);
dt = 0.001;
x_k_1(1) = 2*cos(x_k(5)*dt) * x_k(1) - x_k(2) ;
x_k_1(2) = x_k(1);
x_k_1(3) = 2*cos(x_k(5)*dt) * x_k(3) - x_k(4);
x_k_1(4) = x_k(3);
x_k_1(5) = x_k(5);
 
end

== matlab function RL_sus_quarter_sim/Quarter_sys/Control/Y_1/IFEKF freq bc/Subsystem/MATLAB Function ==
  data: u input; FS_1 input; y output; FS_2 input; FS_3 input
function y = fcn(u,FS_1,FS_2,FS_3)

    if u < FS_1
        y = 3;
    elseif u >= FS_1 && u < FS_2
        y = 1;
    elseif u >= FS_2 && u < FS_3
        y = 2;
    else
        y = 1;
    end
end

== matlab function RL_sus_quarter_sim/Quarter_sys/Control/Y_1/IFEKF freq bc/Subsystem/MATLAB Function2/EKF simple Amp/MATLAB Function ==
  data: gamma input; y output size=[4,4]
function y = fcn(gamma)
% u = [0;0;gamma;1];
u = [0;0;1;gamma];
y = diag(u);
end

== matlab function RL_sus_quarter_sim/Quarter_sys/Control/Y_1/IFEKF freq bc/Subsystem/MATLAB Function2/adaptive IFEKF simple/MATLAB Function ==
  data: x_k input; x_k_1 output
function x_k_1 = IFEKF_tfcn_simp(x_k)
x_k_1 = zeros(5,1);
dt = 0.001;
x_k_1(1) = 2*cos(x_k(5)*dt) * x_k(1) - x_k(2) ;
x_k_1(2) = x_k(1);
x_k_1(3) = 2*cos(x_k(5)*dt) * x_k(3) - x_k(4);
x_k_1(4) = x_k(3);
x_k_1(5) = x_k(5);
 
end

== matlab function RL_sus_quarter_sim/Quarter_sys/Control/Y_1/IFEKF freq bc/Subsystem/MATLAB Function1 ==
  data: u input; FS_1 input; y output; FS_2 input
function y = fcn(u,FS_1,FS_2)

    if u < FS_1
        y = 2;
    elseif u >= FS_1 && u < FS_2
        y = 1;
    else
        y = 1;
    end
end

== matlab function RL_sus_quarter_sim/Quarter_sys/Control/Y_1/IFEKF freq c/Subsystem/MATLAB Function2/EKF simple Amp/MATLAB Function ==
  data: gamma input; y output size=[4,4]
function y = fcn(gamma)
% u = [0;0;gamma;1];
u = [0;0;1;gamma];
y = diag(u);
end

== matlab function RL_sus_quarter_sim/Quarter_sys/Control/Y_1/IFEKF freq c/Subsystem/MATLAB Function2/adaptive IFEKF simple/MATLAB Function ==
  data: x_k input; x_k_1 output
function x_k_1 = IFEKF_tfcn_simp(x_k)
x_k_1 = zeros(5,1);
dt = 0.001;
x_k_1(1) = 2*cos(x_k(5)*dt) * x_k(1) - x_k(2) ;
x_k_1(2) = x_k(1);
x_k_1(3) = 2*cos(x_k(5)*dt) * x_k(3) - x_k(4);
x_k_1(4) = x_k(3);
x_k_1(5) = x_k(5);
 
end

== matlab function RL_sus_quarter_sim/Quarter_sys/Control/Y_1/IFEKF FDC/Subsystem/MATLAB Function ==
  data: u input; y output; FS_2 input; vs input; vdef input; alpha input
function y = fcn(u,FS_2,vs,vdef,alpha)
    % 1skyhook 2add 3cmid

    % if u < FS_1
    %     y = 3;
    % elseif u >= FS_1 && u < FS_2
    %     y = 1;
    % elseif u >= FS_2 && u < FS_3
    %     y = 2;
    % else
    %     y = 1;
    % end
    if fcn1(vs,vdef,alpha) == 1
        y = 1;
    else
        if u < FS_2
            y = 2;
        else
            y = 3;
        end
    end
end

function y = fcn1(vs,vdef,alpha)
cs =1000;
ks = 20000;
ms = 400;

H_alpha = (cs^2*alpha^2+ks^2)/(ms^2*alpha^2);
    if (vdef^2*H_alpha - alpha^2 * vs^2)<=0
            y = 1;
    else
            y = 2;
    end
end

== matlab function RL_sus_quarter_sim/Quarter_sys/Control/Y_1/IFEKF FDC/Subsystem/MATLAB Function2/EKF simple Amp/MATLAB Function ==
  data: gamma input; y output size=[4,4]
function y = fcn(gamma)
% u = [0;0;gamma;1];
u = [0;0;1;gamma];
y = diag(u);
end

== matlab function RL_sus_quarter_sim/Quarter_sys/Control/Y_1/IFEKF FDC/Subsystem/MATLAB Function2/adaptive IFEKF simple/MATLAB Function ==
  data: x_k input; x_k_1 output
function x_k_1 = IFEKF_tfcn_simp(x_k)
x_k_1 = zeros(5,1);
dt = 0.001;
x_k_1(1) = 2*cos(x_k(5)*dt) * x_k(1) - x_k(2) ;
x_k_1(2) = x_k(1);
x_k_1(3) = 2*cos(x_k(5)*dt) * x_k(3) - x_k(4);
x_k_1(4) = x_k(3);
x_k_1(5) = x_k(5);
 
end

== matlab function RL_sus_quarter_sim/Quarter_sys/Control/Y_1/imp_force_RL_model/Subsystem/MATLAB Function2/adaptive IFEKF simple/MATLAB Function ==
  data: x_k input; x_k_1 output
function x_k_1 = IFEKF_tfcn_simp(x_k)
x_k_1 = zeros(5,1);
dt = 0.001;
x_k_1(1) = 2*cos(x_k(5)*dt) * x_k(1) - x_k(2) ;
x_k_1(2) = x_k(1);
x_k_1(3) = 2*cos(x_k(5)*dt) * x_k(3) - x_k(4);
x_k_1(4) = x_k(3);
x_k_1(5) = x_k(5);
 
end

== matlab function RL_sus_quarter_sim/Quarter_sys/Control/Y_1/SH_ADD_new_FS/Modify_SHADD/MATLAB Function ==
  data: y output; vs input; vdef input; alpha input; cs input; ks input; ms input
function y = fcn(vs,vdef,alpha,cs,ks,ms)

    % if u < FS_1
    %     y = 3;
    % elseif u >= FS_1 && u < FS_2
    %     y = 1;
    % elseif u >= FS_2 && u < FS_3
    %     y = 2;
    % else
    %     y = 1;
    % end
    if fcn1(vs,vdef,alpha,cs,ks,ms) == 1
        y = 1;
    else
        y = 2;
    end
end

function y = fcn1(vs,vdef,alpha,cs,ks,ms)
% cs =1000;
% ks = 20000;
% ms = 400;

H_alpha = (cs^2*alpha^2+ks^2)/(ms^2*alpha^2);
    if (vdef^2*H_alpha - alpha^2 * vs^2)<=0
            y = 1;
    else
            y = 0;
    end
end

== matlab function RL_sus_quarter_sim/Quarter_sys/Control/Y_1/SH_ADD/MATLAB Function ==
  data: as input; y output; vs input; vdef input; alpha input; FS output
function [y,FS] = fcn(as,vs,vdef,alpha)
    if (as^2 - alpha^2 * vs^2)<=0
        FS = 1;
        if vs * vdef >0
            y = 1;
        else
            y = 0;
        end
    else
        FS = 2;
        if as * vdef >0
            y = 1;
        else
            y = 0;
        end
    end

end

== matlab function RL_sus_quarter_sim/Quarter_sys/Control/Y_1/IFEKF FDC/Subsystem/MATLAB Function1 ==
  data: u input; y output; FS_2 input; vs input; as input; alpha input
function y = fcn(u,FS_2,vs,as,alpha)
    % 1skyhook 2add 3cmid

    % if u < FS_1
    %     y = 3;
    % elseif u >= FS_1 && u < FS_2
    %     y = 1;
    % elseif u >= FS_2 && u < FS_3
    %     y = 2;
    % else
    %     y = 1;
    % end
    if fcn1(vs,as,alpha) == 1
        y = 1;
    else
        if u < FS_2
            y = 2;
        else
            y = 3;
        end
    end
end

function y = fcn1(vs,as,alpha)
% cs =1000;
% ks = 20000;
% ms = 400;

% H_alpha = (cs^2*alpha^2+ks^2)/(ms^2*alpha^2);
    if (as^2 - alpha^2 * vs^2)<=0
            y = 1;
    else
            y = 2;
    end
end

== matlab function RL_sus_quarter_sim/Quarter_sys/Control/Y_1/SH_ADD_modify/MATLAB Function ==
  data: y output; vs input; vdef input; alpha input; cs input; ks input; ms input
function y = fcn(vs,vdef,alpha,cs,ks,ms)

    % if u < FS_1
    %     y = 3;
    % elseif u >= FS_1 && u < FS_2
    %     y = 1;
    % elseif u >= FS_2 && u < FS_3
    %     y = 2;
    % else
    %     y = 1;
    % end
    if fcn1(vs,vdef,alpha,cs,ks,ms) == 1
        y = 1;
    else
        y = 2;
    end
end

function y = fcn1(vs,vdef,alpha,cs,ks,ms)
% cs =1000;
% ks = 20000;
% ms = 400;

H_alpha = (cs^2*alpha^2+ks^2)/(ms^2*alpha^2);
    if (vdef^2*H_alpha - alpha^2 * vs^2)<=0
            y = 1;
    else
            y = 0;
    end
end

== matlab function RL_sus_quarter_sim/Quarter_sys/Control/Y_1/IFEKF FDC/Subsystem/MATLAB Function2/adaptive IFEKF sdimple_3/MATLAB Function ==
  data: x_k input; x_k_1 output
function x_k_1 = IFEKF_tfcn_simp_3(x_k)
x_k_1 = zeros(3,1);
dt = 0.001;
x_k_1(1) = 2*cos(x_k(3)*dt) * x_k(1) - x_k(2) ;
x_k_1(2) = x_k(1);
% x_k_1(3) = 2*cos(x_k(5)*dt) * x_k(3) - x_k(4);
% x_k_1(4) = x_k(3);
x_k_1(3) = x_k(3);
 
end

== matlab function RL_sus_quarter_sim/Quarter_sys/Control/Y_1/IFEKF FDC/Subsystem/MATLAB Function3 ==
  data: u input; vs input; as input; alpha input; y output; alpha2 input; alpha3 input
function y = fcn(u,vs,as,alpha,alpha2,alpha3)
    % 1skyhook 2add 3cmid

    % if u < FS_1
    %     y = 3;
    % elseif u >= FS_1 && u < FS_2
    %     y = 1;
    % elseif u >= FS_2 && u < FS_3
    %     y = 2;
    % else
    %     y = 1;
    % end
    if fcn1(vs,as,alpha) == 1
        y = 1;
    else
        if u < alpha2 
            y = 2;
        elseif u > alpha3
            y = 2;
        else
            y = 3;
        end
    end
end

function y = fcn1(vs,as,alpha)
% cs =1000;
% ks = 20000;
% ms = 400;

% H_alpha = (cs^2*alpha^2+ks^2)/(ms^2*alpha^2);
    if (as^2 - alpha^2 * vs^2)<=0
            y = 1;
    else
            y = 2;
    end
end

== stateflow chart RL_sus_quarter_sim/Quarter_sys/Control/Y_1/IFEKF freq bkkcc/Subsystem/Chart1 ==
  state L1
    entry:count = 0;
    level = 1;
    during:count = count+1;
    level = 1;
  state L2
    entry:count = 0;
    level = 2;
    during:count = count+1;
    level = 2;
  state L3
    entry:count = 0;
    level = 3;
    during:count = count+1;
    level = 3;
  state L4
    entry:count = 0;
    level = 4;
    during:count = count+1;
    level = 4;
  state L5
    entry:count = 0;
    level = 5;
    during:count = count+1;
    level = 5;
  state L6
    entry:count = 0;
    level = 6;
    during:count = count+1;
    level = 6;
  state L7
    entry:count = 0;
    level = 7;
    during:count = count+1;
    level = 7;
  (default) -> L1
  L1 -> L2 : [freq > (FS1+0.1)&&freq < (FS2-0.1)&&count>=200]
  L6 -> L7 [order 2] : [freq > (FS6+0.1)&&count>=100]
  L2 -> L1 [order 2] : [(freq<(FS1-0.1)&&count>=200)]
  L2 -> L3 [order 1] : [freq > (FS2+0.1)&&freq<(FS3-0.1)&&count>=100]
  L3 -> L4 [order 1] : [freq > (FS3+0.1)&&freq<(FS4-0.1)&&count>=100]
  L4 -> L5 [order 1] : [freq > (FS4+0.1)&&freq<(FS5-0.1)&&count>=100]
  L5 -> L6 [order 2] : [freq > (FS5+0.1)&&freq<(FS6-0.1)&&count>=100]
  L3 -> L2 [order 2] : [freq > (FS1+0.1)&&freq < (FS2-0.1)&&count>=100]
  L7 -> L6 : [freq > (FS5+0.1)&&freq<(FS6-0.1)&&count>=100]
  L5 -> L4 [order 1] : [freq > (FS3+0.1)&&freq<(FS4-0.1)&&count>=100]
  L6 -> L5 [order 1] : [freq > (FS4+0.1)&&freq<(FS5-0.1)&&count>=100]
  L4 -> L3 [order 2] : [freq > (FS2+0.1)&&freq<(FS3-0.1)&&count>=100]
  data: freq input; level output; FS3 constant double =7; count local; FS1 constant double =0.85; FS2 constant double =2.6; FS4 constant double =10; FS5 constant double =12.3; FS6 constant double =13.9

== matlab function RL_sus_quarter_sim/Quarter_sys/Control/Y_1/freq semi/Subsystem/2nd_FS/MATLAB Function1 ==
  data: au input; y output; alpha input; ks input; ms input; cs input
function y = fcn(au,alpha,ks,ms,cs)

y = au^2 * (ks^2 + alpha^2 * cs^2)/((ks-alpha^2*ms)^2 + alpha^2 * cs^2);
end
